simulink model "ship"  (R2021b)
settings: Solver=FixedStepAuto  StartTime=0.0  StopTime=1000  FixedStep=0.05  RelTol=1e-3
settings Model: Creator=simengangstad  LastModifiedBy=simengangstad

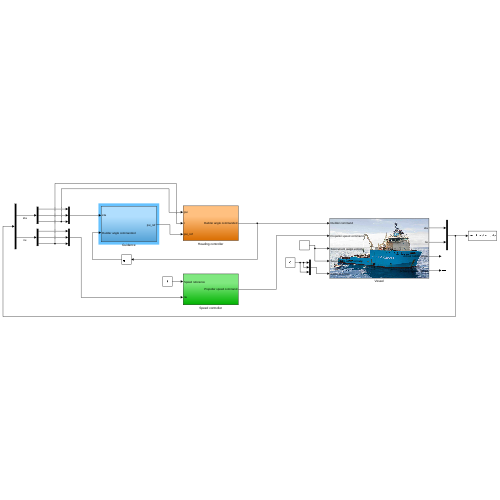
[thumbnail: Simulink's stored preview of the top-level diagram]
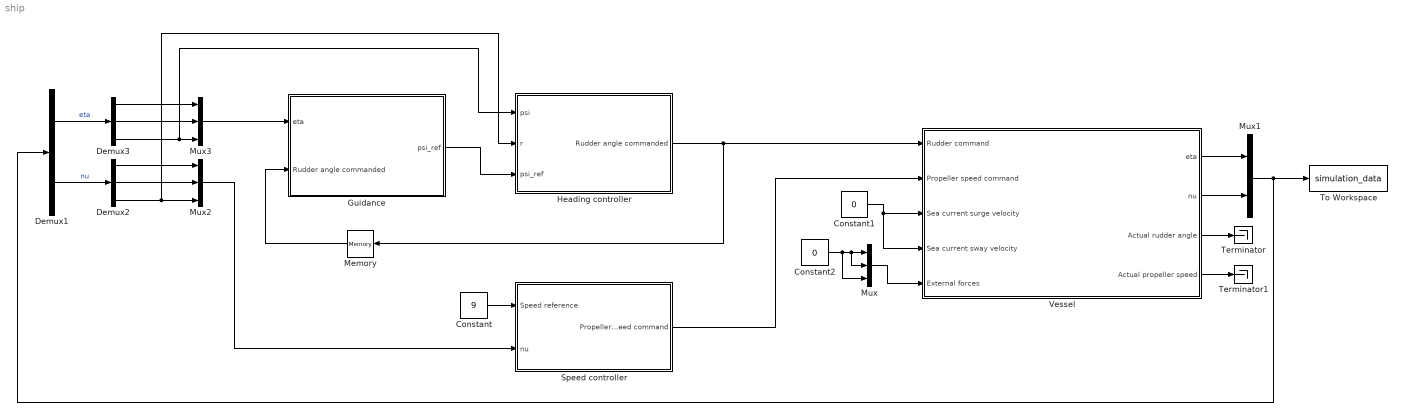
== system ship ==
  Constant : Constant  Value=9
  Constant1 : Constant  Value=0
  Constant2 : Constant  Value=0
  Demux1 : Demux  Outputs=2
  Demux2 : Demux  Outputs=3
  Demux3 : Demux  Outputs=3
  Guidance : Subsystem
  Heading controller : Subsystem
  Memory : Memory
  Mux : Mux  Inputs=3
  Mux1 : Mux  Inputs=2
  Mux2 : Mux  Inputs=3
  Mux3 : Mux  Inputs=3
  Speed controller : Subsystem
  Terminator : Terminator
  Terminator1 : Terminator
  To Workspace : ToWorkspace  VariableName=simulation_data  SaveFormat=Timeseries  SampleTime=-1
  Vessel : Subsystem
      mask Display: image('supply.jpg'); % Use "Edit Image" on toolstrip to change.
  wires:
  Guidance/1(psi_ref) -> Heading controller/3(psi_ref)
  Speed controller/1(Propeller speed command) -> Vessel/2(Propeller speed command)
  Constant/1 -> Speed controller/1(Speed reference)
  Constant1/1 -> Vessel/4(Sea current sway velocity), Vessel/3(Sea current surge velocity)
  Memory/1 -> Guidance/2(Rudder angle commanded)
  Mux/1 -> Vessel/5(External forces)
  Constant2/1 -> Mux/3, Mux/2, Mux/1
  Vessel/1(eta) -> Mux1/1
  Vessel/2(nu) -> Mux1/2
  Mux1/1 -> Demux1/1, To Workspace/1
  Demux2/1 -> Mux2/1
  Demux2/2 -> Mux2/2
  Demux2/3 -> Mux2/3, Heading controller/2(r)
  Demux1/2 -> Demux2/1  "nu"
  Demux3/1 -> Mux3/1
  Demux3/2 -> Mux3/2
  Demux3/3 -> Heading controller/1(psi), Mux3/3
  Demux1/1 -> Demux3/1  "eta"
  Mux2/1 -> Speed controller/2(nu)
  Mux3/1 -> Guidance/1(eta)
  Heading controller/1(Rudder angle commanded) -> Vessel/1(Rudder command), Memory/1
  Vessel/3(Actual rudder angle) -> Terminator/1
  Vessel/4(Actual propeller speed) -> Terminator1/1

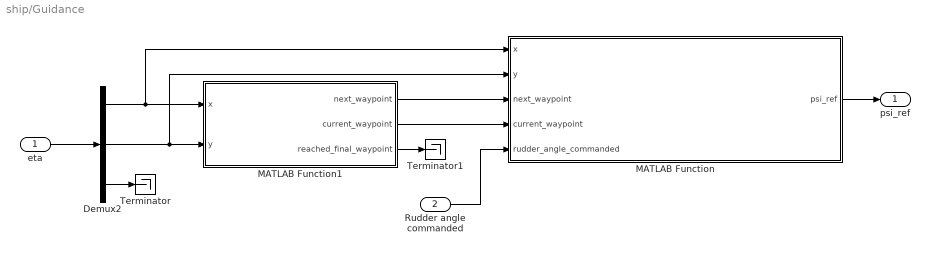
== system ship/Guidance ==
  eta : Inport
  Rudder angle commanded : Inport  Port=2
  Demux2 : Demux  Outputs=3
  MATLAB Function : MATLAB Function  TreatAsAtomicUnit=on
  MATLAB Function1 : MATLAB Function  TreatAsAtomicUnit=on
  Terminator : Terminator
  Terminator1 : Terminator
  psi_ref : Outport
  wires:
  MATLAB Function/1(psi_ref) -> psi_ref/1
  eta/1 -> Demux2/1
  Rudder angle commanded/1 -> MATLAB Function/5(rudder_angle_commanded)
  Demux2/1 -> MATLAB Function/1(x), MATLAB Function1/1(x)
  Demux2/2 -> MATLAB Function/2(y), MATLAB Function1/2(y)
  MATLAB Function1/1(next_waypoint) -> MATLAB Function/3(next_waypoint)
  MATLAB Function1/2(current_waypoint) -> MATLAB Function/4(current_waypoint)
  Demux2/3 -> Terminator/1
  MATLAB Function1/3(reached_final_waypoint) -> Terminator1/1

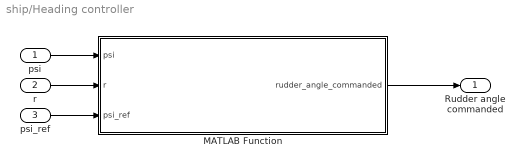
== system ship/Heading controller ==
  psi : Inport
  r : Inport  Port=2
  psi_ref : Inport  Port=3
  MATLAB Function : MATLAB Function  TreatAsAtomicUnit=on
  Rudder angle commanded : Outport
  wires:
  MATLAB Function/1(rudder_angle_commanded) -> Rudder angle commanded/1
  psi_ref/1 -> MATLAB Function/3(psi_ref)
  r/1 -> MATLAB Function/2(r)
  psi/1 -> MATLAB Function/1(psi)

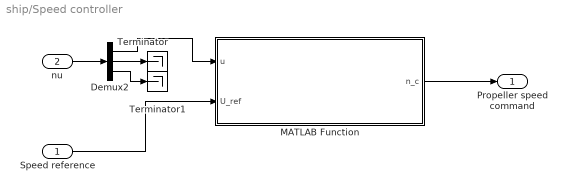
== system ship/Speed controller ==
  Speed reference : Inport
  nu : Inport  Port=2
  Demux2 : Demux  Outputs=3
  MATLAB Function : MATLAB Function  TreatAsAtomicUnit=on
  Terminator : Terminator
  Terminator1 : Terminator
  Propeller speed command : Outport
  wires:
  Demux2/1 -> MATLAB Function/1(u)
  Speed reference/1 -> MATLAB Function/2(U_ref)
  nu/1 -> Demux2/1
  MATLAB Function/1(n_c) -> Propeller speed command/1
  Demux2/2 -> Terminator/1
  Demux2/3 -> Terminator1/1

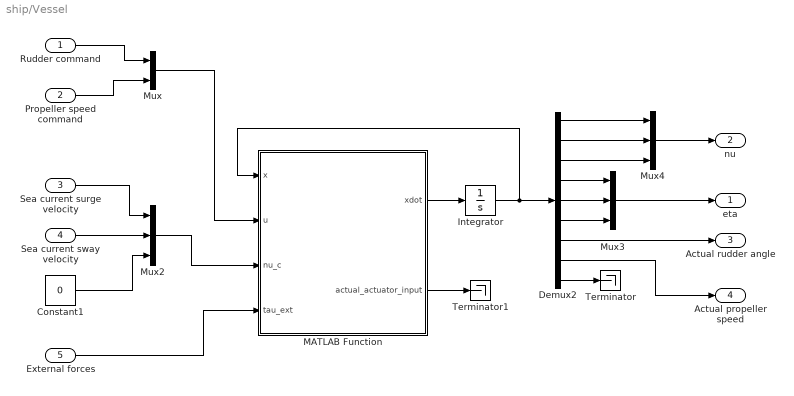
== system ship/Vessel ==
  Rudder command : Inport
  Propeller speed command : Inport  Port=2
  Sea current surge velocity : Inport  Port=3
  Sea current sway velocity : Inport  Port=4
  External forces : Inport  Port=5
  Constant1 : Constant  Value=0
  Demux2 : Demux  Outputs=9
  Integrator : Integrator
  MATLAB Function : MATLAB Function  TreatAsAtomicUnit=on
  Mux : Mux  Inputs=2
  Mux2 : Mux  Inputs=3
  Mux3 : Mux  Inputs=3
  Mux4 : Mux  Inputs=3
  Terminator : Terminator
  Terminator1 : Terminator
  eta : Outport
  nu : Outport  Port=2
  Actual rudder angle : Outport  Port=3
  Actual propeller speed : Outport  Port=4
  wires:
  Demux2/3 -> Mux4/3
  Demux2/7 -> Actual rudder angle/1
  Mux/1 -> MATLAB Function/2(u)
  External forces/1 -> MATLAB Function/4(tau_ext)
  Mux2/1 -> MATLAB Function/3(nu_c)
  Mux4/1 -> nu/1
  MATLAB Function/1(xdot) -> Integrator/1
  Propeller speed command/1 -> Mux/2
  Demux2/4 -> Mux3/1
  Demux2/5 -> Mux3/2
  Sea current surge velocity/1 -> Mux2/1
  Constant1/1 -> Mux2/3
  Sea current sway velocity/1 -> Mux2/2
  Mux3/1 -> eta/1
  Demux2/2 -> Mux4/2
  Demux2/8 -> Actual propeller speed/1
  Demux2/1 -> Mux4/1
  Integrator/1 -> MATLAB Function/1(x), Demux2/1
  Rudder command/1 -> Mux/1
  Demux2/6 -> Mux3/3
  Demux2/9 -> Terminator/1
  MATLAB Function/2(actual_actuator_input) -> Terminator1/1

== matlab function ship/Guidance/MATLAB Function ==
  settings: updateMethod=DISCRETE
  data: x input size=1; y input size=1; next_waypoint input; current_waypoint input; rudder_angle_commanded input size=1; psi_ref output; parameters parameter
function psi_ref = guidance_law(x, y, next_waypoint, current_waypoint, rudder_angle_commanded, parameters)
    % Input:
    % (x, y): Position
    % delta_c: Commanded rudder angle
    % kappa: 
    % parameters: Ship parameters
    %
    % Output:
    % psi_ref: The heading to hold

    persistent y_int
    
    if isempty(y_int)
        y_int = 0;
    end

    % [xk1, yk1, xk, yk, ~] = wp_selector(x, x, parameters.ship.length); 
    [e_y, pi_p] = cross_track_error(next_waypoint(1), ...
                                    next_waypoint(2), ...
                                    current_waypoint(1), ...
                                    current_waypoint(2), ...
                                    x, ...
                                    y);
    [psi_desired, y_int_dot] = ilos_guidance(e_y, ...
                                             pi_p, ...
                                             y_int, ...
                                             parameters.guidance.look_ahead, ...
                                             parameters.guidance.kappa);
    psi_ref = psi_desired;

    % Anti-integrator windup
    if abs(rudder_angle_commanded) <= parameters.rudder.max_angle
        y_int = euler2(y_int_dot, y_int, parameters.simulation.step_size);
    end

== matlab function ship/Vessel/MATLAB Function ==
  data: x input size=9; u input size=2; xdot output size=9; nu_c input size=3; tau_ext input size=3; actual_actuator_input output size=2; parameters parameter
function [xdot, actual_actuator_input] = ship(x, u, nu_c, tau_ext, parameters)
    [xdot, actual_actuator_input] = ship_model(x, u, nu_c, tau_ext, parameters);
end

== matlab function ship/Heading controller/MATLAB Function ==
  settings: updateMethod=DISCRETE  sampleTime=0.05
  data: psi input size=1; r input size=1; psi_ref input size=1; rudder_angle_commanded output size=1; parameters parameter
function rudder_angle_commanded = heading_control(psi, r, psi_ref, parameters)
    % Input: 
    % psi: Heading
    % r: Heading rate
    % psi_ref: Heading reference
    % parameters: Ship parameters
    %
    % rudder_angle_commanded: The desired rudder angle

    persistent psi_ref_x e_psi_int;
    
    if isempty(psi_ref_x)
        psi_ref_x = [0; 0; 0];
    end
    
    if isempty(e_psi_int)
        e_psi_int = 0;
    end

    % The derivative coming from the reference model is the state
    % derivative of the reference model
    psi_ref_x_dot = heading_reference_model(psi_ref_x, psi_ref);

    % We can the extract the desired state for heading (psi)
    % and heading rate (r) from the reference model
    psi_desired = psi_ref_x(1);
    r_desired = psi_ref_x(2);

    % Control law
    e_psi = ssa(psi - psi_desired);
    e_r = ssa(r - r_desired);

    % Now we retrieve the rudder angle command from the heading PID
    rudder_angle_commanded = heading_pid(e_psi, ...
                                         e_r, ...
                                         e_psi_int, ...
                                         parameters.nomoto); 
    
    % Anti-integrator windup
    if abs(rudder_angle_commanded) <= parameters.rudder.max_angle
        e_psi_int = euler2(e_psi, e_psi_int, parameters.simulation.step_size);
    else
        rudder_angle_commanded = parameters.rudder.max_angle ... 
                                 * sign(rudder_angle_commanded);
    end
    
    % Don't care about the integrator windup for the reference model
    psi_ref_x = euler2(psi_ref_x_dot, psi_ref_x, parameters.simulation.step_size);

== matlab function ship/Speed controller/MATLAB Function ==
  settings: updateMethod=DISCRETE  sampleTime=0.05
  data: u input; n_c output; U_ref input; parameters parameter
function n_c = speed_control(u, U_ref, parameters)

    persistent e_u_int

    if isempty(e_u_int)
        e_u_int = 0;
    end

    u_desired = U_ref;
    e_u = u - u_desired;

    % Here n_c is the rps of the motor (n) commanded 
    n_c = speed_pid(u_desired, e_u, e_u_int, parameters);

    e_u_int = euler2(e_u, e_u_int, parameters.simulation.step_size);

== matlab function ship/Guidance/MATLAB Function1 ==
  settings: updateMethod=DISCRETE
  data: x input; next_waypoint output; y input; current_waypoint output; parameters parameter; reached_final_waypoint output
function [next_waypoint, current_waypoint, reached_final_waypoint] = waypoint_selector(x, y, parameters) 
    reached_final_waypoint = 0;
    persistent first k WP_ R_k_1

    if isempty(first)
        WP = load('WP.mat');
        first = 0;
        k = 1;
        WP_ = [WP.WP(1,:), WP.WP(2,:)];
        R_k_1 = 4 * parameters.ship.length;
    end

    n = length(WP_) / 2;            % Number of waypoints
    wpt.x = WP_(1:n);               % North coordinates
    wpt.y = WP_(n+1:2*n);           % East coordinates

    % Choose the correct waypoints
    xk  = wpt.x(k);
    xk1 = wpt.x(k+1);
    yk  = wpt.y(k);
    yk1 = wpt.y(k+1);

    % Update waypoints
    if (xk1 - x)^2 + (yk1 - y)^2 <= R_k_1^2 
        
        if k < n - 1
            k = k + 1;
        else
            reached_final_waypoint = 1;
        end 
    end

    next_waypoint = [xk1, yk1];
    current_waypoint = [xk, yk];
end
